simulink model "rls_test"  (R2018a)
settings: Solver=VariableStepAuto  StartTime=0.0  StopTime=100  RelTol=1e-3
undefined symbols (not defined in the file): atable, atableall, high_speed_Ki, high_speed_Kp, speed_controller_input_limit, station_Ki, station_Kp, T_btde, T_btno, T_delay, utable, utableall, vtable
settings Model: Creator=cidi-xh  LastModifiedBy=cidi-xh

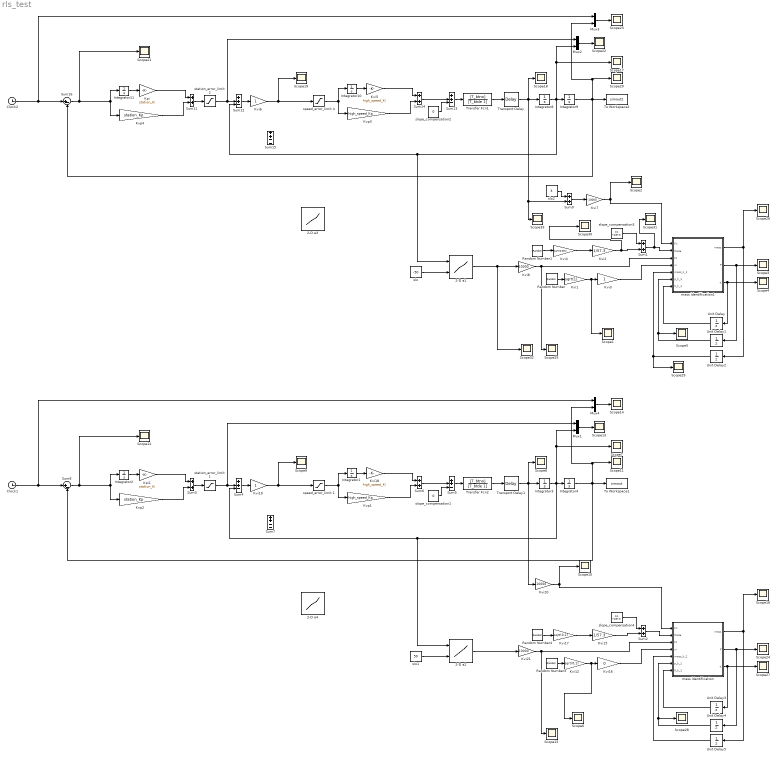
== system rls_test ==
  2-D a1 : Lookup_n-D  BreakpointsForDimension1=vtable  BreakpointsForDimension2=utable  BreakpointsForDimension3=[-60 -50]  Table=atableall  InternalRulePriority=Speed  RndMeth=Simplest  InputSameDT=on
  2-D a2 : Lookup_n-D  BreakpointsForDimension1=vtable  BreakpointsForDimension2=utable  BreakpointsForDimension3=[-60 -50]  Table=atableall  InternalRulePriority=Speed  RndMeth=Simplest  InputSameDT=on
  2-D a3 : Lookup_n-D  BreakpointsForDimension1=vtable  BreakpointsForDimension2=atable  BreakpointsForDimension3=[-60 -50]  Table=utableall  InternalRulePriority=Speed  RndMeth=Simplest  InputSameDT=on
  2-D a4 : Lookup_n-D  BreakpointsForDimension1=vtable  BreakpointsForDimension2=atable  BreakpointsForDimension3=[-60 -50]  Table=utableall  InternalRulePriority=Speed  RndMeth=Simplest  InputSameDT=on
  Clock1 : Clock
  Clock2 : Clock
  Integrator{1..4,8..11} (8 alike) : Integrator
  Kpi : Gain  Gain=station_Ki
  Kpi1 : Gain  Gain=station_Ki
  Kvi1 : Gain  Gain=sqrt(1)
  Kvi12 : Gain  Gain=sqrt(0.1)
  Kvi15 : Gain  Gain=1/57.3
  Kvi16 : Gain  Gain=0
  Kvi17 : Gain  Gain=sqrt(0.1)
  Kvi18 : Gain  Gain=high_speed_Ki
  Kvi19 : Gain
  Kvi2 : Gain  Gain=1/57.3
  Kvi20 : Gain  Gain=10000
  Kvi21 : Gain  Gain=10000
  Kvi3 : Gain
  Kvi4 : Gain  Gain=sqrt(0.001)
  Kvi5 : Gain  Gain=high_speed_Ki
  Kvi6 : Gain
  Kvi7 : Gain  Gain=-10000
  Kvi8 : Gain  Gain=10000
  Kvp1 : Gain  Gain=high_speed_Kp
  Kvp2 : Gain  Gain=station_Kp
  Kvp3 : Gain  Gain=high_speed_Kp
  Kvp4 : Gain  Gain=station_Kp
  Mux{1..4} (4 alike) : Mux  Inputs=2
  Random Number : RandomNumber  SampleTime=0.01
  Random Number1 : RandomNumber  Variance=0.1  SampleTime=0.01
  Random Number3 : RandomNumber  SampleTime=0.01
  Random Number4 : RandomNumber  SampleTime=0.01
  Scope{1..33} (33 alike) : Scope
  Sum{1..3,6,9,11,14} (7 alike) : Sum
  Sum{4..5,12..13} (4 alike) : Sum  Inputs=++-
  Sum15 : Sum  Inputs=++--
  Sum16 : Sum  Inputs=|+-
  Sum7 : Sum  Inputs=++--
  Sum8 : Sum  Inputs=|+-
  To Workspace1 : ToWorkspace  VariableName=simout  SaveFormat=Timeseries  SampleTime=-1
  To Workspace2 : ToWorkspace  VariableName=simout2  SaveFormat=Timeseries  SampleTime=-1
  Transfer Fcn1 : TransferFcn  Numerator=[T_btno]  Denominator=[T_btde 1]
  Transfer Fcn2 : TransferFcn  Numerator=[T_btno]  Denominator=[T_btde 1]
  Transport Delay : TransportDelay  DelayTime=T_delay
  Transport Delay1 : TransportDelay  DelayTime=T_delay
  Unit Delay : UnitDelay  InitialCondition=1  SampleTime=0.01
  Unit Delay1 : UnitDelay  InitialCondition=100000  SampleTime=0.01
  Unit Delay2 : UnitDelay  InitialCondition=30000  SampleTime=0.01
  Unit Delay3 : UnitDelay  InitialCondition=1  SampleTime=0.01
  Unit Delay4 : UnitDelay  InitialCondition=1000000  SampleTime=0.01
  Unit Delay5 : UnitDelay  InitialCondition=50000  SampleTime=0.01
  mass identification : MATLAB Function  TreatAsAtomicUnit=on  SystemSampleTime=0.01
  mass identification1 : MATLAB Function  TreatAsAtomicUnit=on  SystemSampleTime=0.01
  slo : Constant  Value=-50
  slo1 : Constant  Value=50
  slo2 : Constant  Value=3
  slope_compensation1 : Constant  Value=0
  slope_compensation2 : Constant  Value=0
  slope_compensation3 : Constant  Value=0.1 *1/57.3
  slope_compensation4 : Constant  Value=0.1 *1/57.3
  speed_error_limit 1 : Saturate  UpperLimit=speed_controller_input_limit  LowerLimit=-speed_controller_input_limit
  speed_error_limit 4 : Saturate  UpperLimit=speed_controller_input_limit  LowerLimit=-speed_controller_input_limit
  station_error_limit 1 : Saturate  UpperLimit=speed_controller_input_limit  LowerLimit=-speed_controller_input_limit
  station_error_limit 2 : Saturate  UpperLimit=speed_controller_input_limit  LowerLimit=-speed_controller_input_limit
  wires:
  station_error_limit 2/1 -> Sum12/2, Mux2/1
  Integrator11/1 -> Kpi/1
  Integrator8/1 -> Integrator9/1, 2-D a1/1, Sum12/3, Scope17/1, Mux2/2
  Kvi7/1 -> Scope2/1, mass identification1/1(Fc)
  Sum13/1 -> Transfer Fcn1/1
  Mux3/1 -> Scope23/1
  Sum16/1 -> Integrator11/1, Kvp4/1, Scope21/1
  Sum14/1 -> Sum13/2
  Kvi8/1 -> Scope25/1, mass identification1/3(Ft)
  Sum12/1 -> Kvi6/1
  Integrator9/1 -> To Workspace2/1, Scope20/1, Mux3/2, Sum16/2
  Integrator10/1 -> Kvi5/1
  2-D a1/1 -> Scope32/1, Kvi8/1
  Transfer Fcn1/1 -> Transport Delay/1
  Clock2/1 -> Sum16/1, Mux3/1
  Kvp3/1 -> Sum14/2
  slope_compensation2/1 -> Sum13/3
  Kvi5/1 -> Sum14/1
  slo/1 -> 2-D a1/2
  Sum11/1 -> station_error_limit 2/1
  Random Number/1 -> Kvi1/1
  mass identification1/1(mass) -> Unit Delay2/1, Scope26/1
  Kvp4/1 -> Sum11/2
  Kpi/1 -> Sum11/1
  speed_error_limit 4/1 -> Kvp3/1, Integrator10/1
  Kvi6/1 -> speed_error_limit 4/1, Scope19/1
  Mux2/1 -> Scope22/1
  Transport Delay/1 -> Sum9/2, Scope33/1, Integrator8/1, Scope18/1
  Kvi1/1 -> Scope1/1, Kvi3/1
  mass identification1/3(K) -> Unit Delay/1, Scope4/1
  mass identification1/2(P) -> Unit Delay1/1, Scope3/1
  Unit Delay/1 -> mass identification1/7(K_k_1)
  Unit Delay1/1 -> Scope5/1, mass identification1/6(p_k_1)
  Unit Delay2/1 -> Scope29/1, mass identification1/5(mass_k_1)
  Random Number1/1 -> Kvi4/1
  Kvi3/1 -> mass identification1/4(xi)
  Kvi4/1 -> Kvi2/1
  slope_compensation3/1 -> Sum1/1
  Kvi2/1 -> Scope30/1, Sum1/2
  Sum1/1 -> Scope31/1, mass identification1/2(theta)
  Sum2/1 -> mass identification/2(theta)
  Kvi15/1 -> Sum2/2
  slope_compensation4/1 -> Sum2/1
  Kvi17/1 -> Kvi15/1
  Kvi16/1 -> mass identification/4(xi)
  Random Number4/1 -> Kvi17/1
  Unit Delay5/1 -> mass identification/5(mass_k_1)
  Unit Delay4/1 -> mass identification/6(p_k_1), Scope28/1
  Unit Delay3/1 -> mass identification/7(K_k_1)
  mass identification/2(P) -> Scope24/1, Unit Delay4/1
  mass identification/3(K) -> Scope27/1, Unit Delay3/1
  Kvi12/1 -> Kvi16/1, Scope6/1
  Transport Delay1/1 -> Scope8/1, Integrator3/1, Kvi20/1
  Mux1/1 -> Scope13/1
  Kvi19/1 -> Scope9/1, speed_error_limit 1/1
  speed_error_limit 1/1 -> Integrator1/1, Kvp1/1
  Kpi1/1 -> Sum3/1
  Kvp2/1 -> Sum3/2
  mass identification/1(mass) -> Scope16/1, Unit Delay5/1
  Random Number3/1 -> Kvi12/1
  Sum3/1 -> station_error_limit 1/1
  slo1/1 -> 2-D a2/2
  Kvi18/1 -> Sum6/1
  slope_compensation1/1 -> Sum5/3
  Kvp1/1 -> Sum6/2
  Clock1/1 -> Mux4/1, Sum8/1
  Transfer Fcn2/1 -> Transport Delay1/1
  2-D a2/1 -> Kvi21/1
  Integrator1/1 -> Kvi18/1
  Integrator4/1 -> Sum8/2, Mux4/2, Scope11/1, To Workspace1/1
  Sum4/1 -> Kvi19/1
  Kvi21/1 -> mass identification/3(Ft), Scope15/1
  Sum6/1 -> Sum5/2
  Sum8/1 -> Scope12/1, Kvp2/1, Integrator2/1
  Mux4/1 -> Scope14/1
  Sum5/1 -> Transfer Fcn2/1
  Kvi20/1 -> mass identification/1(Fc), Scope10/1
  Integrator3/1 -> Mux1/2, Scope7/1, Sum4/3, 2-D a2/1, Integrator4/1
  Integrator2/1 -> Kpi1/1
  station_error_limit 1/1 -> Mux1/1, Sum4/2
  Sum9/1 -> Kvi7/1
  slo2/1 -> Sum9/1

== matlab function rls_test/mass identification1 ==
  data: mass output; Fc input; theta input; Ft input; xi input; mass_k_1 input; p_k_1 input; K_k_1 input; P output; K output
function [mass,P,K] = fcn(Fc,theta,Ft,xi,mass_k_1,p_k_1,K_k_1)
% Fc = 0;theta = 0;Ft = 0;
na = 1;nb = 1;d = 3; %structure parameters
uk = 0;%initial value of system input
yk = 0;%initial value of system output
L = 1;
g = 9.8;%unit:m/s^2
w = 0.995;
%theta = 0;% slope of the road,unit:degree or rad?

% xi = sqrt(0.1) * randn(L,1);%white noise 
if theta >= 0 
    i = -sin(theta); 
else
    i = sin(theta); 
end
phi = g * i;

Fg = Fc - Ft - xi;
% mass = 0;% initial value of the object to be estimated
% persistent mass_last;
% mass_last = 0;
% P = 10^6 * eye(na - 1 + nb - 1 + 1);
% Fg = phi * m + xi; % y(k) = phi(k)' * theta + xi 标准的最小二乘形式
% mass_data 

% RLS algorithm
K = p_k_1 * phi / (w + phi' * p_k_1 * phi);
% mass = mass_last + K * (Fg - phi' * mass_last);
mass = mass_k_1 + K * (Fg - phi' * mass_k_1);
P =1 / w * (eye(na - 1 + nb - 1 + 1) - K * phi') * p_k_1;

% mass_last = mass;

== matlab function rls_test/mass identification ==
  data: mass output; Fc input; theta input; Ft input; xi input; mass_k_1 input; p_k_1 input; K_k_1 input; P output; K output
function [mass,P,K] = fcn(Fc,theta,Ft,xi,mass_k_1,p_k_1,K_k_1)
% Fc = 0;theta = 0;Ft = 0;
na = 1;nb = 1;d = 3; %structure parameters
uk = 0;%initial value of system input
yk = 0;%initial value of system output
L = 1;
g = 9.8;%unit:m/s^2
w = 1;
%theta = 0;% slope of the road,unit:degree or rad?

% xi = sqrt(0.1) * randn(L,1);%white noise 
i = -sin(theta);
phi = g * i;

Fg = Fc - Ft - xi;
% mass = 0;% initial value of the object to be estimated
% persistent mass_last;
% mass_last = 0;
% P = 10^6 * eye(na - 1 + nb - 1 + 1);
% Fg = phi * m + xi; % y(k) = phi(k)' * theta + xi 标准的最小二乘形式
% mass_data 

% RLS algorithm
K = p_k_1 * phi / (w + phi' * p_k_1 * phi);
% mass = mass_last + K * (Fg - phi' * mass_last);
mass = mass_k_1 + K * (Fg - phi' * mass_k_1);
P =1 / w * (eye(na - 1 + nb - 1 + 1) - K * phi') * p_k_1;

% mass_last = mass;
